simulink model "V.1.0.SystemsmModelling"  (R2020a)
settings: Solver=ode23t  StartTime=0.0  StopTime=2000  MaxStep=2000.0  RelTol=1e-3
values from neighbouring files (symbols this model uses):
  InitialTemp = 300    [Setup.m]
undefined symbols (not defined in the file or in its folder): commanded_mass_flow, compressor_time_constant, condenser_length, copper_density, environment_temperature, evaporator_length, ground_temperature, max_throat_area, max_throat_temperature, min_throat_area, min_throat_temperature, pipe_diameter, pipe_thickness, target_temperature, temperature_delta, u_sat
libraries: fl_lib x208, refrigeration_lib x90, fl_ps_legacy_lib x50, nesl_utility x45
(part 7 of 7)

== system V.1.0.SystemsmModelling/Air Conditioning System/Air Conditioner Model3/Expansion Valve/Valve Control ==
  Min Throat Area : fl_lib/Physical Signals/Sources/PS Constant  constant=min_throat_area
  Min Throat Temperature : fl_lib/Physical Signals/Sources/PS Constant  constant=min_throat_temperature
  PS Add : fl_ps_legacy_lib/Legacy Physical Signals/Functions/PS Add
      settings: SourceProductBaseCode=SS  InternalSimscapePortConfiguration="{\"Bottom\":[],\"Left\":[{\"id\":\"I1\",\"label\":\"\",\"type\":\"input\"},{\"id\":\"I2\",\"label\":\"\",\"type\":\"input\"}],\"Right\":[{\"id\":\"O\",\"label\":\"\",\"type\":\"output\"}],\"Top\":[]}"
  PS Gain : fl_ps_legacy_lib/Legacy Physical Signals/Functions/PS Gain  gain=(max_throat_area - min_throat_area)/(max_throat_temperature - min_throat_temperature)
  PS Saturation : fl_ps_legacy_lib/Legacy Physical Signals/Nonlinear Operators/PS Saturation  upper_limit=max_throat_area  lower_limit=min_throat_area
      settings: SourceProductBaseCode=SS  InternalSimscapePortConfiguration="{\"Bottom\":[],\"Left\":[{\"id\":\"I\",\"label\":\"\",\"type\":\"input\"}],\"Right\":[{\"id\":\"O\",\"label\":\"\",\"type\":\"output\"}],\"Top\":[]}"
  PS Subtract : fl_ps_legacy_lib/Legacy Physical Signals/Functions/PS Subtract
      settings: SourceProductBaseCode=SS
  mm^2 to m^2 : fl_ps_legacy_lib/Legacy Physical Signals/Functions/PS Gain  gain=1e-6
  S : PMIOPort  Side=Left
  T : PMIOPort  Port=2  Side=Right
  connections:
  mm^2 to m^2/RConn1 -- S/RConn1
  PS Saturation/RConn1 -- mm^2 to m^2/LConn1
  PS Subtract/RConn1 -- PS Gain/LConn1
  T/RConn1 -- PS Subtract/LConn1
  PS Add/RConn1 -- PS Saturation/LConn1
  Min Throat Area/RConn1 -- PS Add/LConn1
  Min Throat Temperature/RConn1 -- PS Subtract/LConn2
  PS Gain/RConn1 -- PS Add/LConn2

== system V.1.0.SystemsmModelling/Air Conditioning System/Air Conditioner Model3/Refrigerator Compartment/Environment Temperature ==
  Constant : Constant  Value=environment_temperature
  Ideal Temperature Source : fl_lib/Thermal/Thermal Sources/Controlled Temperature Source
  Simulink-PS Converter : nesl_utility/Simulink-PS Converter  PhysicalDomain=network_engine_domain  SubClassName=ps_input  LeftPortType=input  RightPortType=output  PseudoPeriodic=off  Frequencies=[]  NoiseDistribution=none  NoiseParameters=[]  Unit=K  AffineConversion=off  FilteringAndDerivatives=zero  SimscapeFilterOrder=1  InputFilterTimeConstant=0.001  UdotUserProvided=1
  Thermal Reference : fl_lib/Thermal/Thermal Elements/Thermal Reference
  T : PMIOPort  Side=Left
  wires:
  Constant/1 -> Simulink-PS Converter/1
  connections:
  Ideal Temperature Source/RConn2 -- Thermal Reference/LConn1
  Ideal Temperature Source/RConn1 -- Simulink-PS Converter/RConn1
  Ideal Temperature Source/LConn1 -- T/RConn1

== system V.1.0.SystemsmModelling/Air Conditioning System/Air Conditioner Model3/Refrigerator Compartment/Heat Flow Sensor ==
  Ideal Heat Flow Sensor : fl_lib/Thermal/Thermal Sensors/Heat Flow Rate Sensor
      settings: SourceProductBaseCode=SS
  B : PMIOPort  Side=Right
  A : PMIOPort  Port=2  Side=Left
  connections:
  Ideal Heat Flow Sensor/RConn2 -- B/RConn1
  Ideal Heat Flow Sensor/LConn1 -- A/RConn1

== system V.1.0.SystemsmModelling/Air Conditioning System/Air Conditioner Model3/Refrigerator Compartment/Temperature Sensor ==
  Ideal Temperature Sensor : fl_lib/Thermal/Thermal Sensors/Temperature Sensor
  PS-Simulink Converter : nesl_utility/PS-Simulink Converter  PhysicalDomain=network_engine_domain  SubClassName=ps_output  LeftPortType=input  RightPortType=output  PseudoPeriodic=off  Frequencies=[]  Unit=K  AffineConversion=off
  Thermal Reference : fl_lib/Thermal/Thermal Elements/Thermal Reference
  A : PMIOPort  Side=Left
  T : Outport
  wires:
  PS-Simulink Converter/1 -> T/1
  connections:
  Ideal Temperature Sensor/LConn1 -- A/RConn1
  Thermal Reference/LConn1 -- Ideal Temperature Sensor/RConn1
  PS-Simulink Converter/LConn1 -- Ideal Temperature Sensor/RConn2

== system V.1.0.SystemsmModelling/Air Conditioning System/Air Conditioner Model4/Expansion Valve/Cycle Sensor 4 ==
  Absolute Reference : refrigeration_lib/Absolute Reference  mdot_A_specify=off  mdot_A_priority=High  mdot_A=0 kg/s  mdot_A_nominal_specify=off  mdot_A_nominal_unit=kg/s  mdot_A_nominal_value=1  phi_A_specify=off  phi_A_priority=High  phi_A=0 kW  phi_A_nominal_specify=off  phi_A_nominal_unit=kW  phi_A_nominal_value=1
      settings: InternalSimscapePortConfiguration="{\"Bottom\":[],\"Left\":[{\"id\":\"A\",\"label\":\"\",\"type\":\"refrigeration.refrigeration\"}],\"Right\":[],\"Top\":[]}"
  Pressure And Energy Sensor : refrigeration_lib/Pressure And Energy Sensor  mdot_specify=off  mdot_priority=High  mdot=0 kg/s  mdot_nominal_specify=off  mdot_nominal_unit=kg/s  mdot_nominal_value=1  phi_specify=off  phi_priority=High  phi=0 kW  phi_nominal_specify=off  phi_nominal_unit=kW  phi_nominal_value=1
      settings: InternalSimscapePortConfiguration="{\"Bottom\":[],\"Left\":[{\"id\":\"A\",\"label\":\"A\",\"type\":\"refrigeration.refrigeration\"},{\"id\":\"P\",\"label\":\"P\",\"type\":\"output\"}],\"Right\":[{\"id\":\"B\",\"label\":\"B\",\"type\":\"refrigeration.refrigeration\"},{\"id\":\"U\",\"label\":\"U\",\"type\":\"output\"}],\"Top\":[]}"
  Thermodynamic Properties Sensor : refrigeration_lib/Thermodynamic Properties Sensor  mdot_A_specify=off  mdot_A_priority=High  mdot_A=0 kg/s  mdot_A_nominal_specify=off  mdot_A_nominal_unit=kg/s  mdot_A_nominal_value=1  phi_A_specify=off  phi_A_priority=High  phi_A=0 kW  phi_A_nominal_specify=off  phi_A_nominal_unit=kW  phi_A_nominal_value=1
      settings: InternalSimscapePortConfiguration="{\"Bottom\":[],\"Left\":[{\"id\":\"V\",\"label\":\"V\",\"type\":\"output\"},{\"id\":\"T\",\"label\":\"T\",\"type\":\"output\"},{\"id\":\"X\",\"label\":\"X\",\"type\":\"output\"}],\"Right\":[{\"id\":\"A\",\"label\":\"A\",\"type\":\"refrigeration.refrigeration\"}],\"Top\":[]}"
  A : PMIOPort  Side=Left
  T : PMIOPort  Port=2  Side=Right
  connections:
  Absolute Reference/LConn1 -- Pressure And Energy Sensor/RConn1
  Pressure And Energy Sensor/LConn1 -- A/RConn1 -- Thermodynamic Properties Sensor/RConn1
  T/RConn1 -- Thermodynamic Properties Sensor/LConn2

== system V.1.0.SystemsmModelling/Air Conditioning System/Air Conditioner Model4/Expansion Valve/Mass Flow Sensor ==
  Mass And Energy Flow Sensor : refrigeration_lib/Mass And Energy Flow Sensor  mdot_specify=off  mdot_priority=High  mdot=0 kg/s  mdot_nominal_specify=off  mdot_nominal_unit=kg/s  mdot_nominal_value=1  phi_specify=off  phi_priority=High  phi=0 kW  phi_nominal_specify=off  phi_nominal_unit=kW  phi_nominal_value=1
      settings: InternalSimscapePortConfiguration="{\"Bottom\":[],\"Left\":[{\"id\":\"A\",\"label\":\"A\",\"type\":\"refrigeration.refrigeration\"},{\"id\":\"M\",\"label\":\"M\",\"type\":\"output\"}],\"Right\":[{\"id\":\"B\",\"label\":\"B\",\"type\":\"refrigeration.refrigeration\"},{\"id\":\"E\",\"label\":\"E\",\"type\":\"output\"}],\"Top\":[]}"
  B : PMIOPort  Side=Right
  A : PMIOPort  Port=2  Side=Left
  connections:
  Mass And Energy Flow Sensor/RConn1 -- B/RConn1
  Mass And Energy Flow Sensor/LConn1 -- A/RConn1

== system V.1.0.SystemsmModelling/Air Conditioning System/Air Conditioner Model4/Expansion Valve/Valve Control ==
  Min Throat Area : fl_lib/Physical Signals/Sources/PS Constant  constant=min_throat_area
  Min Throat Temperature : fl_lib/Physical Signals/Sources/PS Constant  constant=min_throat_temperature
  PS Add : fl_ps_legacy_lib/Legacy Physical Signals/Functions/PS Add
      settings: SourceProductBaseCode=SS  InternalSimscapePortConfiguration="{\"Bottom\":[],\"Left\":[{\"id\":\"I1\",\"label\":\"\",\"type\":\"input\"},{\"id\":\"I2\",\"label\":\"\",\"type\":\"input\"}],\"Right\":[{\"id\":\"O\",\"label\":\"\",\"type\":\"output\"}],\"Top\":[]}"
  PS Gain : fl_ps_legacy_lib/Legacy Physical Signals/Functions/PS Gain  gain=(max_throat_area - min_throat_area)/(max_throat_temperature - min_throat_temperature)
  PS Saturation : fl_ps_legacy_lib/Legacy Physical Signals/Nonlinear Operators/PS Saturation  upper_limit=max_throat_area  lower_limit=min_throat_area
      settings: SourceProductBaseCode=SS  InternalSimscapePortConfiguration="{\"Bottom\":[],\"Left\":[{\"id\":\"I\",\"label\":\"\",\"type\":\"input\"}],\"Right\":[{\"id\":\"O\",\"label\":\"\",\"type\":\"output\"}],\"Top\":[]}"
  PS Subtract : fl_ps_legacy_lib/Legacy Physical Signals/Functions/PS Subtract
      settings: SourceProductBaseCode=SS
  mm^2 to m^2 : fl_ps_legacy_lib/Legacy Physical Signals/Functions/PS Gain  gain=1e-6
  S : PMIOPort  Side=Left
  T : PMIOPort  Port=2  Side=Right
  connections:
  mm^2 to m^2/RConn1 -- S/RConn1
  PS Saturation/RConn1 -- mm^2 to m^2/LConn1
  PS Subtract/RConn1 -- PS Gain/LConn1
  T/RConn1 -- PS Subtract/LConn1
  PS Add/RConn1 -- PS Saturation/LConn1
  Min Throat Area/RConn1 -- PS Add/LConn1
  Min Throat Temperature/RConn1 -- PS Subtract/LConn2
  PS Gain/RConn1 -- PS Add/LConn2

== system V.1.0.SystemsmModelling/Air Conditioning System/Air Conditioner Model4/Refrigerator Compartment/Environment Temperature ==
  Constant : Constant  Value=environment_temperature
  Ideal Temperature Source : fl_lib/Thermal/Thermal Sources/Controlled Temperature Source
  Simulink-PS Converter : nesl_utility/Simulink-PS Converter  PhysicalDomain=network_engine_domain  SubClassName=ps_input  LeftPortType=input  RightPortType=output  PseudoPeriodic=off  Frequencies=[]  NoiseDistribution=none  NoiseParameters=[]  Unit=K  AffineConversion=off  FilteringAndDerivatives=zero  SimscapeFilterOrder=1  InputFilterTimeConstant=0.001  UdotUserProvided=1
  Thermal Reference : fl_lib/Thermal/Thermal Elements/Thermal Reference
  T : PMIOPort  Side=Left
  wires:
  Constant/1 -> Simulink-PS Converter/1
  connections:
  Ideal Temperature Source/RConn2 -- Thermal Reference/LConn1
  Ideal Temperature Source/RConn1 -- Simulink-PS Converter/RConn1
  Ideal Temperature Source/LConn1 -- T/RConn1

== system V.1.0.SystemsmModelling/Air Conditioning System/Air Conditioner Model4/Refrigerator Compartment/Heat Flow Sensor ==
  Ideal Heat Flow Sensor : fl_lib/Thermal/Thermal Sensors/Heat Flow Rate Sensor
      settings: SourceProductBaseCode=SS
  B : PMIOPort  Side=Right
  A : PMIOPort  Port=2  Side=Left
  connections:
  Ideal Heat Flow Sensor/RConn2 -- B/RConn1
  Ideal Heat Flow Sensor/LConn1 -- A/RConn1

== system V.1.0.SystemsmModelling/Air Conditioning System/Air Conditioner Model4/Refrigerator Compartment/Temperature Sensor ==
  Ideal Temperature Sensor : fl_lib/Thermal/Thermal Sensors/Temperature Sensor
  PS-Simulink Converter : nesl_utility/PS-Simulink Converter  PhysicalDomain=network_engine_domain  SubClassName=ps_output  LeftPortType=input  RightPortType=output  PseudoPeriodic=off  Frequencies=[]  Unit=K  AffineConversion=off
  Thermal Reference : fl_lib/Thermal/Thermal Elements/Thermal Reference
  A : PMIOPort  Side=Left
  T : Outport
  wires:
  PS-Simulink Converter/1 -> T/1
  connections:
  Ideal Temperature Sensor/LConn1 -- A/RConn1
  Thermal Reference/LConn1 -- Ideal Temperature Sensor/RConn1
  PS-Simulink Converter/LConn1 -- Ideal Temperature Sensor/RConn2

== system V.1.0.SystemsmModelling/Air Conditioning System/Air Conditioner Model5/Expansion Valve/Cycle Sensor 4 ==
  Absolute Reference : refrigeration_lib/Absolute Reference  mdot_A_specify=off  mdot_A_priority=High  mdot_A=0 kg/s  mdot_A_nominal_specify=off  mdot_A_nominal_unit=kg/s  mdot_A_nominal_value=1  phi_A_specify=off  phi_A_priority=High  phi_A=0 kW  phi_A_nominal_specify=off  phi_A_nominal_unit=kW  phi_A_nominal_value=1
      settings: InternalSimscapePortConfiguration="{\"Bottom\":[],\"Left\":[{\"id\":\"A\",\"label\":\"\",\"type\":\"refrigeration.refrigeration\"}],\"Right\":[],\"Top\":[]}"
  Pressure And Energy Sensor : refrigeration_lib/Pressure And Energy Sensor  mdot_specify=off  mdot_priority=High  mdot=0 kg/s  mdot_nominal_specify=off  mdot_nominal_unit=kg/s  mdot_nominal_value=1  phi_specify=off  phi_priority=High  phi=0 kW  phi_nominal_specify=off  phi_nominal_unit=kW  phi_nominal_value=1
      settings: InternalSimscapePortConfiguration="{\"Bottom\":[],\"Left\":[{\"id\":\"A\",\"label\":\"A\",\"type\":\"refrigeration.refrigeration\"},{\"id\":\"P\",\"label\":\"P\",\"type\":\"output\"}],\"Right\":[{\"id\":\"B\",\"label\":\"B\",\"type\":\"refrigeration.refrigeration\"},{\"id\":\"U\",\"label\":\"U\",\"type\":\"output\"}],\"Top\":[]}"
  Thermodynamic Properties Sensor : refrigeration_lib/Thermodynamic Properties Sensor  mdot_A_specify=off  mdot_A_priority=High  mdot_A=0 kg/s  mdot_A_nominal_specify=off  mdot_A_nominal_unit=kg/s  mdot_A_nominal_value=1  phi_A_specify=off  phi_A_priority=High  phi_A=0 kW  phi_A_nominal_specify=off  phi_A_nominal_unit=kW  phi_A_nominal_value=1
      settings: InternalSimscapePortConfiguration="{\"Bottom\":[],\"Left\":[{\"id\":\"V\",\"label\":\"V\",\"type\":\"output\"},{\"id\":\"T\",\"label\":\"T\",\"type\":\"output\"},{\"id\":\"X\",\"label\":\"X\",\"type\":\"output\"}],\"Right\":[{\"id\":\"A\",\"label\":\"A\",\"type\":\"refrigeration.refrigeration\"}],\"Top\":[]}"
  A : PMIOPort  Side=Left
  T : PMIOPort  Port=2  Side=Right
  connections:
  Absolute Reference/LConn1 -- Pressure And Energy Sensor/RConn1
  Pressure And Energy Sensor/LConn1 -- A/RConn1 -- Thermodynamic Properties Sensor/RConn1
  T/RConn1 -- Thermodynamic Properties Sensor/LConn2

== system V.1.0.SystemsmModelling/Air Conditioning System/Air Conditioner Model5/Expansion Valve/Mass Flow Sensor ==
  Mass And Energy Flow Sensor : refrigeration_lib/Mass And Energy Flow Sensor  mdot_specify=off  mdot_priority=High  mdot=0 kg/s  mdot_nominal_specify=off  mdot_nominal_unit=kg/s  mdot_nominal_value=1  phi_specify=off  phi_priority=High  phi=0 kW  phi_nominal_specify=off  phi_nominal_unit=kW  phi_nominal_value=1
      settings: InternalSimscapePortConfiguration="{\"Bottom\":[],\"Left\":[{\"id\":\"A\",\"label\":\"A\",\"type\":\"refrigeration.refrigeration\"},{\"id\":\"M\",\"label\":\"M\",\"type\":\"output\"}],\"Right\":[{\"id\":\"B\",\"label\":\"B\",\"type\":\"refrigeration.refrigeration\"},{\"id\":\"E\",\"label\":\"E\",\"type\":\"output\"}],\"Top\":[]}"
  B : PMIOPort  Side=Right
  A : PMIOPort  Port=2  Side=Left
  connections:
  Mass And Energy Flow Sensor/RConn1 -- B/RConn1
  Mass And Energy Flow Sensor/LConn1 -- A/RConn1

== system V.1.0.SystemsmModelling/Air Conditioning System/Air Conditioner Model5/Expansion Valve/Valve Control ==
  Min Throat Area : fl_lib/Physical Signals/Sources/PS Constant  constant=min_throat_area
  Min Throat Temperature : fl_lib/Physical Signals/Sources/PS Constant  constant=min_throat_temperature
  PS Add : fl_ps_legacy_lib/Legacy Physical Signals/Functions/PS Add
      settings: SourceProductBaseCode=SS  InternalSimscapePortConfiguration="{\"Bottom\":[],\"Left\":[{\"id\":\"I1\",\"label\":\"\",\"type\":\"input\"},{\"id\":\"I2\",\"label\":\"\",\"type\":\"input\"}],\"Right\":[{\"id\":\"O\",\"label\":\"\",\"type\":\"output\"}],\"Top\":[]}"
  PS Gain : fl_ps_legacy_lib/Legacy Physical Signals/Functions/PS Gain  gain=(max_throat_area - min_throat_area)/(max_throat_temperature - min_throat_temperature)
  PS Saturation : fl_ps_legacy_lib/Legacy Physical Signals/Nonlinear Operators/PS Saturation  upper_limit=max_throat_area  lower_limit=min_throat_area
      settings: SourceProductBaseCode=SS  InternalSimscapePortConfiguration="{\"Bottom\":[],\"Left\":[{\"id\":\"I\",\"label\":\"\",\"type\":\"input\"}],\"Right\":[{\"id\":\"O\",\"label\":\"\",\"type\":\"output\"}],\"Top\":[]}"
  PS Subtract : fl_ps_legacy_lib/Legacy Physical Signals/Functions/PS Subtract
      settings: SourceProductBaseCode=SS
  mm^2 to m^2 : fl_ps_legacy_lib/Legacy Physical Signals/Functions/PS Gain  gain=1e-6
  S : PMIOPort  Side=Left
  T : PMIOPort  Port=2  Side=Right
  connections:
  mm^2 to m^2/RConn1 -- S/RConn1
  PS Saturation/RConn1 -- mm^2 to m^2/LConn1
  PS Subtract/RConn1 -- PS Gain/LConn1
  T/RConn1 -- PS Subtract/LConn1
  PS Add/RConn1 -- PS Saturation/LConn1
  Min Throat Area/RConn1 -- PS Add/LConn1
  Min Throat Temperature/RConn1 -- PS Subtract/LConn2
  PS Gain/RConn1 -- PS Add/LConn2

== system V.1.0.SystemsmModelling/Air Conditioning System/Air Conditioner Model5/Refrigerator Compartment/Environment Temperature ==
  Constant : Constant  Value=environment_temperature
  Ideal Temperature Source : fl_lib/Thermal/Thermal Sources/Controlled Temperature Source
  Simulink-PS Converter : nesl_utility/Simulink-PS Converter  PhysicalDomain=network_engine_domain  SubClassName=ps_input  LeftPortType=input  RightPortType=output  PseudoPeriodic=off  Frequencies=[]  NoiseDistribution=none  NoiseParameters=[]  Unit=K  AffineConversion=off  FilteringAndDerivatives=zero  SimscapeFilterOrder=1  InputFilterTimeConstant=0.001  UdotUserProvided=1
  Thermal Reference : fl_lib/Thermal/Thermal Elements/Thermal Reference
  T : PMIOPort  Side=Left
  wires:
  Constant/1 -> Simulink-PS Converter/1
  connections:
  Ideal Temperature Source/RConn2 -- Thermal Reference/LConn1
  Ideal Temperature Source/RConn1 -- Simulink-PS Converter/RConn1
  Ideal Temperature Source/LConn1 -- T/RConn1

== system V.1.0.SystemsmModelling/Air Conditioning System/Air Conditioner Model5/Refrigerator Compartment/Heat Flow Sensor ==
  Ideal Heat Flow Sensor : fl_lib/Thermal/Thermal Sensors/Heat Flow Rate Sensor
      settings: SourceProductBaseCode=SS
  B : PMIOPort  Side=Right
  A : PMIOPort  Port=2  Side=Left
  connections:
  Ideal Heat Flow Sensor/RConn2 -- B/RConn1
  Ideal Heat Flow Sensor/LConn1 -- A/RConn1

== system V.1.0.SystemsmModelling/Air Conditioning System/Air Conditioner Model5/Refrigerator Compartment/Temperature Sensor ==
  Ideal Temperature Sensor : fl_lib/Thermal/Thermal Sensors/Temperature Sensor
  PS-Simulink Converter : nesl_utility/PS-Simulink Converter  PhysicalDomain=network_engine_domain  SubClassName=ps_output  LeftPortType=input  RightPortType=output  PseudoPeriodic=off  Frequencies=[]  Unit=K  AffineConversion=off
  Thermal Reference : fl_lib/Thermal/Thermal Elements/Thermal Reference
  A : PMIOPort  Side=Left
  T : Outport
  wires:
  PS-Simulink Converter/1 -> T/1
  connections:
  Ideal Temperature Sensor/LConn1 -- A/RConn1
  Thermal Reference/LConn1 -- Ideal Temperature Sensor/RConn1
  PS-Simulink Converter/LConn1 -- Ideal Temperature Sensor/RConn2

== system V.1.0.SystemsmModelling/Air Conditioning System/Air Conditioner Model6/Expansion Valve/Cycle Sensor 4 ==
  Absolute Reference : refrigeration_lib/Absolute Reference  mdot_A_specify=off  mdot_A_priority=High  mdot_A=0 kg/s  mdot_A_nominal_specify=off  mdot_A_nominal_unit=kg/s  mdot_A_nominal_value=1  phi_A_specify=off  phi_A_priority=High  phi_A=0 kW  phi_A_nominal_specify=off  phi_A_nominal_unit=kW  phi_A_nominal_value=1
      settings: InternalSimscapePortConfiguration="{\"Bottom\":[],\"Left\":[{\"id\":\"A\",\"label\":\"\",\"type\":\"refrigeration.refrigeration\"}],\"Right\":[],\"Top\":[]}"
  Pressure And Energy Sensor : refrigeration_lib/Pressure And Energy Sensor  mdot_specify=off  mdot_priority=High  mdot=0 kg/s  mdot_nominal_specify=off  mdot_nominal_unit=kg/s  mdot_nominal_value=1  phi_specify=off  phi_priority=High  phi=0 kW  phi_nominal_specify=off  phi_nominal_unit=kW  phi_nominal_value=1
      settings: InternalSimscapePortConfiguration="{\"Bottom\":[],\"Left\":[{\"id\":\"A\",\"label\":\"A\",\"type\":\"refrigeration.refrigeration\"},{\"id\":\"P\",\"label\":\"P\",\"type\":\"output\"}],\"Right\":[{\"id\":\"B\",\"label\":\"B\",\"type\":\"refrigeration.refrigeration\"},{\"id\":\"U\",\"label\":\"U\",\"type\":\"output\"}],\"Top\":[]}"
  Thermodynamic Properties Sensor : refrigeration_lib/Thermodynamic Properties Sensor  mdot_A_specify=off  mdot_A_priority=High  mdot_A=0 kg/s  mdot_A_nominal_specify=off  mdot_A_nominal_unit=kg/s  mdot_A_nominal_value=1  phi_A_specify=off  phi_A_priority=High  phi_A=0 kW  phi_A_nominal_specify=off  phi_A_nominal_unit=kW  phi_A_nominal_value=1
      settings: InternalSimscapePortConfiguration="{\"Bottom\":[],\"Left\":[{\"id\":\"V\",\"label\":\"V\",\"type\":\"output\"},{\"id\":\"T\",\"label\":\"T\",\"type\":\"output\"},{\"id\":\"X\",\"label\":\"X\",\"type\":\"output\"}],\"Right\":[{\"id\":\"A\",\"label\":\"A\",\"type\":\"refrigeration.refrigeration\"}],\"Top\":[]}"
  A : PMIOPort  Side=Left
  T : PMIOPort  Port=2  Side=Right
  connections:
  Absolute Reference/LConn1 -- Pressure And Energy Sensor/RConn1
  Pressure And Energy Sensor/LConn1 -- A/RConn1 -- Thermodynamic Properties Sensor/RConn1
  T/RConn1 -- Thermodynamic Properties Sensor/LConn2

== system V.1.0.SystemsmModelling/Air Conditioning System/Air Conditioner Model6/Expansion Valve/Mass Flow Sensor ==
  Mass And Energy Flow Sensor : refrigeration_lib/Mass And Energy Flow Sensor  mdot_specify=off  mdot_priority=High  mdot=0 kg/s  mdot_nominal_specify=off  mdot_nominal_unit=kg/s  mdot_nominal_value=1  phi_specify=off  phi_priority=High  phi=0 kW  phi_nominal_specify=off  phi_nominal_unit=kW  phi_nominal_value=1
      settings: InternalSimscapePortConfiguration="{\"Bottom\":[],\"Left\":[{\"id\":\"A\",\"label\":\"A\",\"type\":\"refrigeration.refrigeration\"},{\"id\":\"M\",\"label\":\"M\",\"type\":\"output\"}],\"Right\":[{\"id\":\"B\",\"label\":\"B\",\"type\":\"refrigeration.refrigeration\"},{\"id\":\"E\",\"label\":\"E\",\"type\":\"output\"}],\"Top\":[]}"
  B : PMIOPort  Side=Right
  A : PMIOPort  Port=2  Side=Left
  connections:
  Mass And Energy Flow Sensor/RConn1 -- B/RConn1
  Mass And Energy Flow Sensor/LConn1 -- A/RConn1

== system V.1.0.SystemsmModelling/Air Conditioning System/Air Conditioner Model6/Expansion Valve/Valve Control ==
  Min Throat Area : fl_lib/Physical Signals/Sources/PS Constant  constant=min_throat_area
  Min Throat Temperature : fl_lib/Physical Signals/Sources/PS Constant  constant=min_throat_temperature
  PS Add : fl_ps_legacy_lib/Legacy Physical Signals/Functions/PS Add
      settings: SourceProductBaseCode=SS  InternalSimscapePortConfiguration="{\"Bottom\":[],\"Left\":[{\"id\":\"I1\",\"label\":\"\",\"type\":\"input\"},{\"id\":\"I2\",\"label\":\"\",\"type\":\"input\"}],\"Right\":[{\"id\":\"O\",\"label\":\"\",\"type\":\"output\"}],\"Top\":[]}"
  PS Gain : fl_ps_legacy_lib/Legacy Physical Signals/Functions/PS Gain  gain=(max_throat_area - min_throat_area)/(max_throat_temperature - min_throat_temperature)
  PS Saturation : fl_ps_legacy_lib/Legacy Physical Signals/Nonlinear Operators/PS Saturation  upper_limit=max_throat_area  lower_limit=min_throat_area
      settings: SourceProductBaseCode=SS  InternalSimscapePortConfiguration="{\"Bottom\":[],\"Left\":[{\"id\":\"I\",\"label\":\"\",\"type\":\"input\"}],\"Right\":[{\"id\":\"O\",\"label\":\"\",\"type\":\"output\"}],\"Top\":[]}"
  PS Subtract : fl_ps_legacy_lib/Legacy Physical Signals/Functions/PS Subtract
      settings: SourceProductBaseCode=SS
  mm^2 to m^2 : fl_ps_legacy_lib/Legacy Physical Signals/Functions/PS Gain  gain=1e-6
  S : PMIOPort  Side=Left
  T : PMIOPort  Port=2  Side=Right
  connections:
  mm^2 to m^2/RConn1 -- S/RConn1
  PS Saturation/RConn1 -- mm^2 to m^2/LConn1
  PS Subtract/RConn1 -- PS Gain/LConn1
  T/RConn1 -- PS Subtract/LConn1
  PS Add/RConn1 -- PS Saturation/LConn1
  Min Throat Area/RConn1 -- PS Add/LConn1
  Min Throat Temperature/RConn1 -- PS Subtract/LConn2
  PS Gain/RConn1 -- PS Add/LConn2

== system V.1.0.SystemsmModelling/Air Conditioning System/Air Conditioner Model6/Refrigerator Compartment/Environment Temperature ==
  Constant : Constant  Value=environment_temperature
  Ideal Temperature Source : fl_lib/Thermal/Thermal Sources/Controlled Temperature Source
  Simulink-PS Converter : nesl_utility/Simulink-PS Converter  PhysicalDomain=network_engine_domain  SubClassName=ps_input  LeftPortType=input  RightPortType=output  PseudoPeriodic=off  Frequencies=[]  NoiseDistribution=none  NoiseParameters=[]  Unit=K  AffineConversion=off  FilteringAndDerivatives=zero  SimscapeFilterOrder=1  InputFilterTimeConstant=0.001  UdotUserProvided=1
  Thermal Reference : fl_lib/Thermal/Thermal Elements/Thermal Reference
  T : PMIOPort  Side=Left
  wires:
  Constant/1 -> Simulink-PS Converter/1
  connections:
  Ideal Temperature Source/RConn2 -- Thermal Reference/LConn1
  Ideal Temperature Source/RConn1 -- Simulink-PS Converter/RConn1
  Ideal Temperature Source/LConn1 -- T/RConn1

== system V.1.0.SystemsmModelling/Air Conditioning System/Air Conditioner Model6/Refrigerator Compartment/Heat Flow Sensor ==
  Ideal Heat Flow Sensor : fl_lib/Thermal/Thermal Sensors/Heat Flow Rate Sensor
      settings: SourceProductBaseCode=SS
  B : PMIOPort  Side=Right
  A : PMIOPort  Port=2  Side=Left
  connections:
  Ideal Heat Flow Sensor/RConn2 -- B/RConn1
  Ideal Heat Flow Sensor/LConn1 -- A/RConn1

== system V.1.0.SystemsmModelling/Air Conditioning System/Air Conditioner Model6/Refrigerator Compartment/Temperature Sensor ==
  Ideal Temperature Sensor : fl_lib/Thermal/Thermal Sensors/Temperature Sensor
  PS-Simulink Converter : nesl_utility/PS-Simulink Converter  PhysicalDomain=network_engine_domain  SubClassName=ps_output  LeftPortType=input  RightPortType=output  PseudoPeriodic=off  Frequencies=[]  Unit=K  AffineConversion=off
  Thermal Reference : fl_lib/Thermal/Thermal Elements/Thermal Reference
  A : PMIOPort  Side=Left
  T : Outport
  wires:
  PS-Simulink Converter/1 -> T/1
  connections:
  Ideal Temperature Sensor/LConn1 -- A/RConn1
  Thermal Reference/LConn1 -- Ideal Temperature Sensor/RConn1
  PS-Simulink Converter/LConn1 -- Ideal Temperature Sensor/RConn2

== system V.1.0.SystemsmModelling/Air Conditioning System/Air Conditioner Model7/Expansion Valve/Cycle Sensor 4 ==
  Absolute Reference : refrigeration_lib/Absolute Reference  mdot_A_specify=off  mdot_A_priority=High  mdot_A=0 kg/s  mdot_A_nominal_specify=off  mdot_A_nominal_unit=kg/s  mdot_A_nominal_value=1  phi_A_specify=off  phi_A_priority=High  phi_A=0 kW  phi_A_nominal_specify=off  phi_A_nominal_unit=kW  phi_A_nominal_value=1
      settings: InternalSimscapePortConfiguration="{\"Bottom\":[],\"Left\":[{\"id\":\"A\",\"label\":\"\",\"type\":\"refrigeration.refrigeration\"}],\"Right\":[],\"Top\":[]}"
  Pressure And Energy Sensor : refrigeration_lib/Pressure And Energy Sensor  mdot_specify=off  mdot_priority=High  mdot=0 kg/s  mdot_nominal_specify=off  mdot_nominal_unit=kg/s  mdot_nominal_value=1  phi_specify=off  phi_priority=High  phi=0 kW  phi_nominal_specify=off  phi_nominal_unit=kW  phi_nominal_value=1
      settings: InternalSimscapePortConfiguration="{\"Bottom\":[],\"Left\":[{\"id\":\"A\",\"label\":\"A\",\"type\":\"refrigeration.refrigeration\"},{\"id\":\"P\",\"label\":\"P\",\"type\":\"output\"}],\"Right\":[{\"id\":\"B\",\"label\":\"B\",\"type\":\"refrigeration.refrigeration\"},{\"id\":\"U\",\"label\":\"U\",\"type\":\"output\"}],\"Top\":[]}"
  Thermodynamic Properties Sensor : refrigeration_lib/Thermodynamic Properties Sensor  mdot_A_specify=off  mdot_A_priority=High  mdot_A=0 kg/s  mdot_A_nominal_specify=off  mdot_A_nominal_unit=kg/s  mdot_A_nominal_value=1  phi_A_specify=off  phi_A_priority=High  phi_A=0 kW  phi_A_nominal_specify=off  phi_A_nominal_unit=kW  phi_A_nominal_value=1
      settings: InternalSimscapePortConfiguration="{\"Bottom\":[],\"Left\":[{\"id\":\"V\",\"label\":\"V\",\"type\":\"output\"},{\"id\":\"T\",\"label\":\"T\",\"type\":\"output\"},{\"id\":\"X\",\"label\":\"X\",\"type\":\"output\"}],\"Right\":[{\"id\":\"A\",\"label\":\"A\",\"type\":\"refrigeration.refrigeration\"}],\"Top\":[]}"
  A : PMIOPort  Side=Left
  T : PMIOPort  Port=2  Side=Right
  connections:
  Absolute Reference/LConn1 -- Pressure And Energy Sensor/RConn1
  Pressure And Energy Sensor/LConn1 -- A/RConn1 -- Thermodynamic Properties Sensor/RConn1
  T/RConn1 -- Thermodynamic Properties Sensor/LConn2

== system V.1.0.SystemsmModelling/Air Conditioning System/Air Conditioner Model7/Expansion Valve/Mass Flow Sensor ==
  Mass And Energy Flow Sensor : refrigeration_lib/Mass And Energy Flow Sensor  mdot_specify=off  mdot_priority=High  mdot=0 kg/s  mdot_nominal_specify=off  mdot_nominal_unit=kg/s  mdot_nominal_value=1  phi_specify=off  phi_priority=High  phi=0 kW  phi_nominal_specify=off  phi_nominal_unit=kW  phi_nominal_value=1
      settings: InternalSimscapePortConfiguration="{\"Bottom\":[],\"Left\":[{\"id\":\"A\",\"label\":\"A\",\"type\":\"refrigeration.refrigeration\"},{\"id\":\"M\",\"label\":\"M\",\"type\":\"output\"}],\"Right\":[{\"id\":\"B\",\"label\":\"B\",\"type\":\"refrigeration.refrigeration\"},{\"id\":\"E\",\"label\":\"E\",\"type\":\"output\"}],\"Top\":[]}"
  B : PMIOPort  Side=Right
  A : PMIOPort  Port=2  Side=Left
  connections:
  Mass And Energy Flow Sensor/RConn1 -- B/RConn1
  Mass And Energy Flow Sensor/LConn1 -- A/RConn1

== system V.1.0.SystemsmModelling/Air Conditioning System/Air Conditioner Model7/Expansion Valve/Valve Control ==
  Min Throat Area : fl_lib/Physical Signals/Sources/PS Constant  constant=min_throat_area
  Min Throat Temperature : fl_lib/Physical Signals/Sources/PS Constant  constant=min_throat_temperature
  PS Add : fl_ps_legacy_lib/Legacy Physical Signals/Functions/PS Add
      settings: SourceProductBaseCode=SS  InternalSimscapePortConfiguration="{\"Bottom\":[],\"Left\":[{\"id\":\"I1\",\"label\":\"\",\"type\":\"input\"},{\"id\":\"I2\",\"label\":\"\",\"type\":\"input\"}],\"Right\":[{\"id\":\"O\",\"label\":\"\",\"type\":\"output\"}],\"Top\":[]}"
  PS Gain : fl_ps_legacy_lib/Legacy Physical Signals/Functions/PS Gain  gain=(max_throat_area - min_throat_area)/(max_throat_temperature - min_throat_temperature)
  PS Saturation : fl_ps_legacy_lib/Legacy Physical Signals/Nonlinear Operators/PS Saturation  upper_limit=max_throat_area  lower_limit=min_throat_area
      settings: SourceProductBaseCode=SS  InternalSimscapePortConfiguration="{\"Bottom\":[],\"Left\":[{\"id\":\"I\",\"label\":\"\",\"type\":\"input\"}],\"Right\":[{\"id\":\"O\",\"label\":\"\",\"type\":\"output\"}],\"Top\":[]}"
  PS Subtract : fl_ps_legacy_lib/Legacy Physical Signals/Functions/PS Subtract
      settings: SourceProductBaseCode=SS
  mm^2 to m^2 : fl_ps_legacy_lib/Legacy Physical Signals/Functions/PS Gain  gain=1e-6
  S : PMIOPort  Side=Left
  T : PMIOPort  Port=2  Side=Right
  connections:
  mm^2 to m^2/RConn1 -- S/RConn1
  PS Saturation/RConn1 -- mm^2 to m^2/LConn1
  PS Subtract/RConn1 -- PS Gain/LConn1
  T/RConn1 -- PS Subtract/LConn1
  PS Add/RConn1 -- PS Saturation/LConn1
  Min Throat Area/RConn1 -- PS Add/LConn1
  Min Throat Temperature/RConn1 -- PS Subtract/LConn2
  PS Gain/RConn1 -- PS Add/LConn2

== system V.1.0.SystemsmModelling/Air Conditioning System/Air Conditioner Model7/Refrigerator Compartment/Environment Temperature ==
  Constant : Constant  Value=environment_temperature
  Ideal Temperature Source : fl_lib/Thermal/Thermal Sources/Controlled Temperature Source
  Simulink-PS Converter : nesl_utility/Simulink-PS Converter  PhysicalDomain=network_engine_domain  SubClassName=ps_input  LeftPortType=input  RightPortType=output  PseudoPeriodic=off  Frequencies=[]  NoiseDistribution=none  NoiseParameters=[]  Unit=K  AffineConversion=off  FilteringAndDerivatives=zero  SimscapeFilterOrder=1  InputFilterTimeConstant=0.001  UdotUserProvided=1
  Thermal Reference : fl_lib/Thermal/Thermal Elements/Thermal Reference
  T : PMIOPort  Side=Left
  wires:
  Constant/1 -> Simulink-PS Converter/1
  connections:
  Ideal Temperature Source/RConn2 -- Thermal Reference/LConn1
  Ideal Temperature Source/RConn1 -- Simulink-PS Converter/RConn1
  Ideal Temperature Source/LConn1 -- T/RConn1

== system V.1.0.SystemsmModelling/Air Conditioning System/Air Conditioner Model7/Refrigerator Compartment/Heat Flow Sensor ==
  Ideal Heat Flow Sensor : fl_lib/Thermal/Thermal Sensors/Heat Flow Rate Sensor
      settings: SourceProductBaseCode=SS
  B : PMIOPort  Side=Right
  A : PMIOPort  Port=2  Side=Left
  connections:
  Ideal Heat Flow Sensor/RConn2 -- B/RConn1
  Ideal Heat Flow Sensor/LConn1 -- A/RConn1

== system V.1.0.SystemsmModelling/Air Conditioning System/Air Conditioner Model7/Refrigerator Compartment/Temperature Sensor ==
  Ideal Temperature Sensor : fl_lib/Thermal/Thermal Sensors/Temperature Sensor
  PS-Simulink Converter : nesl_utility/PS-Simulink Converter  PhysicalDomain=network_engine_domain  SubClassName=ps_output  LeftPortType=input  RightPortType=output  PseudoPeriodic=off  Frequencies=[]  Unit=K  AffineConversion=off
  Thermal Reference : fl_lib/Thermal/Thermal Elements/Thermal Reference
  A : PMIOPort  Side=Left
  T : Outport
  wires:
  PS-Simulink Converter/1 -> T/1
  connections:
  Ideal Temperature Sensor/LConn1 -- A/RConn1
  Thermal Reference/LConn1 -- Ideal Temperature Sensor/RConn1
  PS-Simulink Converter/LConn1 -- Ideal Temperature Sensor/RConn2

== system V.1.0.SystemsmModelling/Air Conditioning System/Air Conditioner Model8/Expansion Valve/Cycle Sensor 4 ==
  Absolute Reference : refrigeration_lib/Absolute Reference  mdot_A_specify=off  mdot_A_priority=High  mdot_A=0 kg/s  mdot_A_nominal_specify=off  mdot_A_nominal_unit=kg/s  mdot_A_nominal_value=1  phi_A_specify=off  phi_A_priority=High  phi_A=0 kW  phi_A_nominal_specify=off  phi_A_nominal_unit=kW  phi_A_nominal_value=1
      settings: InternalSimscapePortConfiguration="{\"Bottom\":[],\"Left\":[{\"id\":\"A\",\"label\":\"\",\"type\":\"refrigeration.refrigeration\"}],\"Right\":[],\"Top\":[]}"
  Pressure And Energy Sensor : refrigeration_lib/Pressure And Energy Sensor  mdot_specify=off  mdot_priority=High  mdot=0 kg/s  mdot_nominal_specify=off  mdot_nominal_unit=kg/s  mdot_nominal_value=1  phi_specify=off  phi_priority=High  phi=0 kW  phi_nominal_specify=off  phi_nominal_unit=kW  phi_nominal_value=1
      settings: InternalSimscapePortConfiguration="{\"Bottom\":[],\"Left\":[{\"id\":\"A\",\"label\":\"A\",\"type\":\"refrigeration.refrigeration\"},{\"id\":\"P\",\"label\":\"P\",\"type\":\"output\"}],\"Right\":[{\"id\":\"B\",\"label\":\"B\",\"type\":\"refrigeration.refrigeration\"},{\"id\":\"U\",\"label\":\"U\",\"type\":\"output\"}],\"Top\":[]}"
  Thermodynamic Properties Sensor : refrigeration_lib/Thermodynamic Properties Sensor  mdot_A_specify=off  mdot_A_priority=High  mdot_A=0 kg/s  mdot_A_nominal_specify=off  mdot_A_nominal_unit=kg/s  mdot_A_nominal_value=1  phi_A_specify=off  phi_A_priority=High  phi_A=0 kW  phi_A_nominal_specify=off  phi_A_nominal_unit=kW  phi_A_nominal_value=1
      settings: InternalSimscapePortConfiguration="{\"Bottom\":[],\"Left\":[{\"id\":\"V\",\"label\":\"V\",\"type\":\"output\"},{\"id\":\"T\",\"label\":\"T\",\"type\":\"output\"},{\"id\":\"X\",\"label\":\"X\",\"type\":\"output\"}],\"Right\":[{\"id\":\"A\",\"label\":\"A\",\"type\":\"refrigeration.refrigeration\"}],\"Top\":[]}"
  A : PMIOPort  Side=Left
  T : PMIOPort  Port=2  Side=Right
  connections:
  Absolute Reference/LConn1 -- Pressure And Energy Sensor/RConn1
  Pressure And Energy Sensor/LConn1 -- A/RConn1 -- Thermodynamic Properties Sensor/RConn1
  T/RConn1 -- Thermodynamic Properties Sensor/LConn2

== system V.1.0.SystemsmModelling/Air Conditioning System/Air Conditioner Model8/Expansion Valve/Mass Flow Sensor ==
  Mass And Energy Flow Sensor : refrigeration_lib/Mass And Energy Flow Sensor  mdot_specify=off  mdot_priority=High  mdot=0 kg/s  mdot_nominal_specify=off  mdot_nominal_unit=kg/s  mdot_nominal_value=1  phi_specify=off  phi_priority=High  phi=0 kW  phi_nominal_specify=off  phi_nominal_unit=kW  phi_nominal_value=1
      settings: InternalSimscapePortConfiguration="{\"Bottom\":[],\"Left\":[{\"id\":\"A\",\"label\":\"A\",\"type\":\"refrigeration.refrigeration\"},{\"id\":\"M\",\"label\":\"M\",\"type\":\"output\"}],\"Right\":[{\"id\":\"B\",\"label\":\"B\",\"type\":\"refrigeration.refrigeration\"},{\"id\":\"E\",\"label\":\"E\",\"type\":\"output\"}],\"Top\":[]}"
  B : PMIOPort  Side=Right
  A : PMIOPort  Port=2  Side=Left
  connections:
  Mass And Energy Flow Sensor/RConn1 -- B/RConn1
  Mass And Energy Flow Sensor/LConn1 -- A/RConn1

== system V.1.0.SystemsmModelling/Air Conditioning System/Air Conditioner Model8/Expansion Valve/Valve Control ==
  Min Throat Area : fl_lib/Physical Signals/Sources/PS Constant  constant=min_throat_area
  Min Throat Temperature : fl_lib/Physical Signals/Sources/PS Constant  constant=min_throat_temperature
  PS Add : fl_ps_legacy_lib/Legacy Physical Signals/Functions/PS Add
      settings: SourceProductBaseCode=SS  InternalSimscapePortConfiguration="{\"Bottom\":[],\"Left\":[{\"id\":\"I1\",\"label\":\"\",\"type\":\"input\"},{\"id\":\"I2\",\"label\":\"\",\"type\":\"input\"}],\"Right\":[{\"id\":\"O\",\"label\":\"\",\"type\":\"output\"}],\"Top\":[]}"
  PS Gain : fl_ps_legacy_lib/Legacy Physical Signals/Functions/PS Gain  gain=(max_throat_area - min_throat_area)/(max_throat_temperature - min_throat_temperature)
  PS Saturation : fl_ps_legacy_lib/Legacy Physical Signals/Nonlinear Operators/PS Saturation  upper_limit=max_throat_area  lower_limit=min_throat_area
      settings: SourceProductBaseCode=SS  InternalSimscapePortConfiguration="{\"Bottom\":[],\"Left\":[{\"id\":\"I\",\"label\":\"\",\"type\":\"input\"}],\"Right\":[{\"id\":\"O\",\"label\":\"\",\"type\":\"output\"}],\"Top\":[]}"
  PS Subtract : fl_ps_legacy_lib/Legacy Physical Signals/Functions/PS Subtract
      settings: SourceProductBaseCode=SS
  mm^2 to m^2 : fl_ps_legacy_lib/Legacy Physical Signals/Functions/PS Gain  gain=1e-6
  S : PMIOPort  Side=Left
  T : PMIOPort  Port=2  Side=Right
  connections:
  mm^2 to m^2/RConn1 -- S/RConn1
  PS Saturation/RConn1 -- mm^2 to m^2/LConn1
  PS Subtract/RConn1 -- PS Gain/LConn1
  T/RConn1 -- PS Subtract/LConn1
  PS Add/RConn1 -- PS Saturation/LConn1
  Min Throat Area/RConn1 -- PS Add/LConn1
  Min Throat Temperature/RConn1 -- PS Subtract/LConn2
  PS Gain/RConn1 -- PS Add/LConn2

== system V.1.0.SystemsmModelling/Air Conditioning System/Air Conditioner Model8/Refrigerator Compartment/Environment Temperature ==
  Constant : Constant  Value=environment_temperature
  Ideal Temperature Source : fl_lib/Thermal/Thermal Sources/Controlled Temperature Source
  Simulink-PS Converter : nesl_utility/Simulink-PS Converter  PhysicalDomain=network_engine_domain  SubClassName=ps_input  LeftPortType=input  RightPortType=output  PseudoPeriodic=off  Frequencies=[]  NoiseDistribution=none  NoiseParameters=[]  Unit=K  AffineConversion=off  FilteringAndDerivatives=zero  SimscapeFilterOrder=1  InputFilterTimeConstant=0.001  UdotUserProvided=1
  Thermal Reference : fl_lib/Thermal/Thermal Elements/Thermal Reference
  T : PMIOPort  Side=Left
  wires:
  Constant/1 -> Simulink-PS Converter/1
  connections:
  Ideal Temperature Source/RConn2 -- Thermal Reference/LConn1
  Ideal Temperature Source/RConn1 -- Simulink-PS Converter/RConn1
  Ideal Temperature Source/LConn1 -- T/RConn1

== system V.1.0.SystemsmModelling/Air Conditioning System/Air Conditioner Model8/Refrigerator Compartment/Heat Flow Sensor ==
  Ideal Heat Flow Sensor : fl_lib/Thermal/Thermal Sensors/Heat Flow Rate Sensor
      settings: SourceProductBaseCode=SS
  B : PMIOPort  Side=Right
  A : PMIOPort  Port=2  Side=Left
  connections:
  Ideal Heat Flow Sensor/RConn2 -- B/RConn1
  Ideal Heat Flow Sensor/LConn1 -- A/RConn1

== system V.1.0.SystemsmModelling/Air Conditioning System/Air Conditioner Model8/Refrigerator Compartment/Temperature Sensor ==
  Ideal Temperature Sensor : fl_lib/Thermal/Thermal Sensors/Temperature Sensor
  PS-Simulink Converter : nesl_utility/PS-Simulink Converter  PhysicalDomain=network_engine_domain  SubClassName=ps_output  LeftPortType=input  RightPortType=output  PseudoPeriodic=off  Frequencies=[]  Unit=K  AffineConversion=off
  Thermal Reference : fl_lib/Thermal/Thermal Elements/Thermal Reference
  A : PMIOPort  Side=Left
  T : Outport
  wires:
  PS-Simulink Converter/1 -> T/1
  connections:
  Ideal Temperature Sensor/LConn1 -- A/RConn1
  Thermal Reference/LConn1 -- Ideal Temperature Sensor/RConn1
  PS-Simulink Converter/LConn1 -- Ideal Temperature Sensor/RConn2

== system V.1.0.SystemsmModelling/Air Conditioning System/Air Conditioner Model9/Expansion Valve/Cycle Sensor 4 ==
  Absolute Reference : refrigeration_lib/Absolute Reference  mdot_A_specify=off  mdot_A_priority=High  mdot_A=0 kg/s  mdot_A_nominal_specify=off  mdot_A_nominal_unit=kg/s  mdot_A_nominal_value=1  phi_A_specify=off  phi_A_priority=High  phi_A=0 kW  phi_A_nominal_specify=off  phi_A_nominal_unit=kW  phi_A_nominal_value=1
      settings: InternalSimscapePortConfiguration="{\"Bottom\":[],\"Left\":[{\"id\":\"A\",\"label\":\"\",\"type\":\"refrigeration.refrigeration\"}],\"Right\":[],\"Top\":[]}"
  Pressure And Energy Sensor : refrigeration_lib/Pressure And Energy Sensor  mdot_specify=off  mdot_priority=High  mdot=0 kg/s  mdot_nominal_specify=off  mdot_nominal_unit=kg/s  mdot_nominal_value=1  phi_specify=off  phi_priority=High  phi=0 kW  phi_nominal_specify=off  phi_nominal_unit=kW  phi_nominal_value=1
      settings: InternalSimscapePortConfiguration="{\"Bottom\":[],\"Left\":[{\"id\":\"A\",\"label\":\"A\",\"type\":\"refrigeration.refrigeration\"},{\"id\":\"P\",\"label\":\"P\",\"type\":\"output\"}],\"Right\":[{\"id\":\"B\",\"label\":\"B\",\"type\":\"refrigeration.refrigeration\"},{\"id\":\"U\",\"label\":\"U\",\"type\":\"output\"}],\"Top\":[]}"
  Thermodynamic Properties Sensor : refrigeration_lib/Thermodynamic Properties Sensor  mdot_A_specify=off  mdot_A_priority=High  mdot_A=0 kg/s  mdot_A_nominal_specify=off  mdot_A_nominal_unit=kg/s  mdot_A_nominal_value=1  phi_A_specify=off  phi_A_priority=High  phi_A=0 kW  phi_A_nominal_specify=off  phi_A_nominal_unit=kW  phi_A_nominal_value=1
      settings: InternalSimscapePortConfiguration="{\"Bottom\":[],\"Left\":[{\"id\":\"V\",\"label\":\"V\",\"type\":\"output\"},{\"id\":\"T\",\"label\":\"T\",\"type\":\"output\"},{\"id\":\"X\",\"label\":\"X\",\"type\":\"output\"}],\"Right\":[{\"id\":\"A\",\"label\":\"A\",\"type\":\"refrigeration.refrigeration\"}],\"Top\":[]}"
  A : PMIOPort  Side=Left
  T : PMIOPort  Port=2  Side=Right
  connections:
  Absolute Reference/LConn1 -- Pressure And Energy Sensor/RConn1
  Pressure And Energy Sensor/LConn1 -- A/RConn1 -- Thermodynamic Properties Sensor/RConn1
  T/RConn1 -- Thermodynamic Properties Sensor/LConn2

== system V.1.0.SystemsmModelling/Air Conditioning System/Air Conditioner Model9/Expansion Valve/Mass Flow Sensor ==
  Mass And Energy Flow Sensor : refrigeration_lib/Mass And Energy Flow Sensor  mdot_specify=off  mdot_priority=High  mdot=0 kg/s  mdot_nominal_specify=off  mdot_nominal_unit=kg/s  mdot_nominal_value=1  phi_specify=off  phi_priority=High  phi=0 kW  phi_nominal_specify=off  phi_nominal_unit=kW  phi_nominal_value=1
      settings: InternalSimscapePortConfiguration="{\"Bottom\":[],\"Left\":[{\"id\":\"A\",\"label\":\"A\",\"type\":\"refrigeration.refrigeration\"},{\"id\":\"M\",\"label\":\"M\",\"type\":\"output\"}],\"Right\":[{\"id\":\"B\",\"label\":\"B\",\"type\":\"refrigeration.refrigeration\"},{\"id\":\"E\",\"label\":\"E\",\"type\":\"output\"}],\"Top\":[]}"
  B : PMIOPort  Side=Right
  A : PMIOPort  Port=2  Side=Left
  connections:
  Mass And Energy Flow Sensor/RConn1 -- B/RConn1
  Mass And Energy Flow Sensor/LConn1 -- A/RConn1

== system V.1.0.SystemsmModelling/Air Conditioning System/Air Conditioner Model9/Expansion Valve/Valve Control ==
  Min Throat Area : fl_lib/Physical Signals/Sources/PS Constant  constant=min_throat_area
  Min Throat Temperature : fl_lib/Physical Signals/Sources/PS Constant  constant=min_throat_temperature
  PS Add : fl_ps_legacy_lib/Legacy Physical Signals/Functions/PS Add
      settings: SourceProductBaseCode=SS  InternalSimscapePortConfiguration="{\"Bottom\":[],\"Left\":[{\"id\":\"I1\",\"label\":\"\",\"type\":\"input\"},{\"id\":\"I2\",\"label\":\"\",\"type\":\"input\"}],\"Right\":[{\"id\":\"O\",\"label\":\"\",\"type\":\"output\"}],\"Top\":[]}"
  PS Gain : fl_ps_legacy_lib/Legacy Physical Signals/Functions/PS Gain  gain=(max_throat_area - min_throat_area)/(max_throat_temperature - min_throat_temperature)
  PS Saturation : fl_ps_legacy_lib/Legacy Physical Signals/Nonlinear Operators/PS Saturation  upper_limit=max_throat_area  lower_limit=min_throat_area
      settings: SourceProductBaseCode=SS  InternalSimscapePortConfiguration="{\"Bottom\":[],\"Left\":[{\"id\":\"I\",\"label\":\"\",\"type\":\"input\"}],\"Right\":[{\"id\":\"O\",\"label\":\"\",\"type\":\"output\"}],\"Top\":[]}"
  PS Subtract : fl_ps_legacy_lib/Legacy Physical Signals/Functions/PS Subtract
      settings: SourceProductBaseCode=SS
  mm^2 to m^2 : fl_ps_legacy_lib/Legacy Physical Signals/Functions/PS Gain  gain=1e-6
  S : PMIOPort  Side=Left
  T : PMIOPort  Port=2  Side=Right
  connections:
  mm^2 to m^2/RConn1 -- S/RConn1
  PS Saturation/RConn1 -- mm^2 to m^2/LConn1
  PS Subtract/RConn1 -- PS Gain/LConn1
  T/RConn1 -- PS Subtract/LConn1
  PS Add/RConn1 -- PS Saturation/LConn1
  Min Throat Area/RConn1 -- PS Add/LConn1
  Min Throat Temperature/RConn1 -- PS Subtract/LConn2
  PS Gain/RConn1 -- PS Add/LConn2

== system V.1.0.SystemsmModelling/Air Conditioning System/Air Conditioner Model9/Refrigerator Compartment/Environment Temperature ==
  Constant : Constant  Value=environment_temperature
  Ideal Temperature Source : fl_lib/Thermal/Thermal Sources/Controlled Temperature Source
  Simulink-PS Converter : nesl_utility/Simulink-PS Converter  PhysicalDomain=network_engine_domain  SubClassName=ps_input  LeftPortType=input  RightPortType=output  PseudoPeriodic=off  Frequencies=[]  NoiseDistribution=none  NoiseParameters=[]  Unit=K  AffineConversion=off  FilteringAndDerivatives=zero  SimscapeFilterOrder=1  InputFilterTimeConstant=0.001  UdotUserProvided=1
  Thermal Reference : fl_lib/Thermal/Thermal Elements/Thermal Reference
  T : PMIOPort  Side=Left
  wires:
  Constant/1 -> Simulink-PS Converter/1
  connections:
  Ideal Temperature Source/RConn2 -- Thermal Reference/LConn1
  Ideal Temperature Source/RConn1 -- Simulink-PS Converter/RConn1
  Ideal Temperature Source/LConn1 -- T/RConn1

== system V.1.0.SystemsmModelling/Air Conditioning System/Air Conditioner Model9/Refrigerator Compartment/Heat Flow Sensor ==
  Ideal Heat Flow Sensor : fl_lib/Thermal/Thermal Sensors/Heat Flow Rate Sensor
      settings: SourceProductBaseCode=SS
  B : PMIOPort  Side=Right
  A : PMIOPort  Port=2  Side=Left
  connections:
  Ideal Heat Flow Sensor/RConn2 -- B/RConn1
  Ideal Heat Flow Sensor/LConn1 -- A/RConn1

== system V.1.0.SystemsmModelling/Air Conditioning System/Air Conditioner Model9/Refrigerator Compartment/Temperature Sensor ==
  Ideal Temperature Sensor : fl_lib/Thermal/Thermal Sensors/Temperature Sensor
  PS-Simulink Converter : nesl_utility/PS-Simulink Converter  PhysicalDomain=network_engine_domain  SubClassName=ps_output  LeftPortType=input  RightPortType=output  PseudoPeriodic=off  Frequencies=[]  Unit=K  AffineConversion=off
  Thermal Reference : fl_lib/Thermal/Thermal Elements/Thermal Reference
  A : PMIOPort  Side=Left
  T : Outport
  wires:
  PS-Simulink Converter/1 -> T/1
  connections:
  Ideal Temperature Sensor/LConn1 -- A/RConn1
  Thermal Reference/LConn1 -- Ideal Temperature Sensor/RConn1
  PS-Simulink Converter/LConn1 -- Ideal Temperature Sensor/RConn2
